simulink model "MCU_VoltLoopCal"  (R2022b)
settings: Solver=FixedStepDiscrete  StartTime=0.0  StopTime=10.0  FixedStep=0.001  RelTol=1e-3
values from neighbouring files (symbols this model uses):
  UDQ_LIMIT_ABS = 1.2    [MCU_VoltLoopCal.sldd]    (also in MCU_VoltLoopCal_objects.m = Simulink.Parameter)
  VOLTLOOP_KI = 0.1    [MCU_VoltLoopCal.sldd]    (also in MCU_VoltLoopCal_objects.m = Simulink.Parameter)
  VOLTLOOP_KP = 0.15    [MCU_VoltLoopCal.sldd]    (also in MCU_VoltLoopCal_objects.m = Simulink.Parameter)
undefined symbols (not defined in the file or in its folder): cCurrentLoopMode, cTorqueLoopMode, ParamCfg_CommandSource_u16, ParamCfg_CurrentPolarCoordinates_u16, ParamCfg_IqMax_u16, ParamCfg_MotorLsd_u16, ParamCfg_RotorFlux_u16, ParamCfg_Vc1Enable_u16, ParamCfg_VdqDest_u16, ParamCfg_WeakIdMax_u16, TESTBED
libraries: simulink x10, YS_UserDefined_Library x2
settings Model: DataDictionary=MCU_VoltLoopCal.sldd  Creator=ZYH  LastModifiedBy=ZYH
settings OptimizationCC: DefaultParameterBehavior=Inlined  EnhancedBackFolding=on  PassReuseOutputArgsAs=Individual arguments  ZeroExternalMemoryAtStartup=off  ZeroInternalMemoryAtStartup=off  OptimizeBlockOrder=speed  DifferentSizesBufferReuse=on  OptimizationCustomize=off  EfficientTunableParamExpr=on
settings DebuggingCC: ParameterTunabilityLossMsg=error
settings SFSimCC: MATLABDynamicMemAlloc=off
settings RTWCC: Description=Embedded Coder  SystemTargetFile=ert.tlc  GenCodeOnly=on  TemplateMakefile=ert_default_tmf
settings CodeAppCC: ForceParamTrailComments=on  IgnoreCustomStorageClasses=off  OperatorAnnotations=on  SimulinkDataObjDesc=on  SFDataObjDesc=on  InsertBlockDesc=on
settings ERTTargetCC: TargetLangStandard=C99 (ISO)  GenerateSampleERTMain=on  InlinedParameterPlacement=NonHierarchical  ERTCustomFileTemplate=example_file_process.tlc

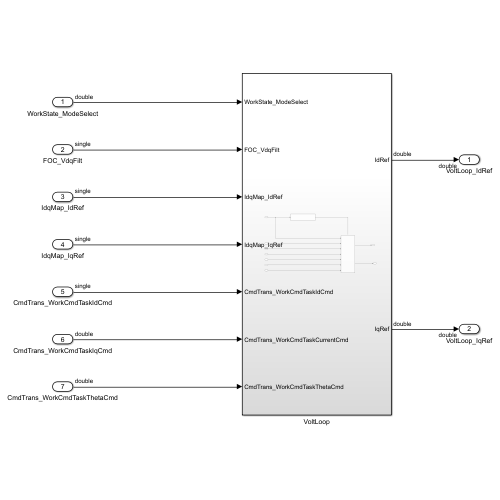
[thumbnail: Simulink's stored preview of the top-level diagram]
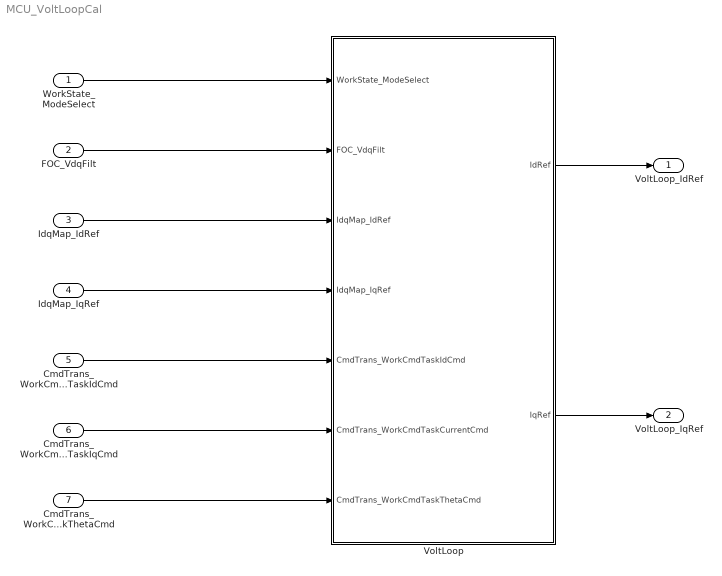
== system MCU_VoltLoopCal ==
  WorkState_ModeSelect : Inport
  FOC_VdqFilt : Inport  Port=2
  IdqMap_IdRef : Inport  Port=3
  IdqMap_IqRef : Inport  Port=4
  CmdTrans_WorkCmdTaskIdCmd : Inport  Port=5
  CmdTrans_WorkCmdTaskIqCmd : Inport  Port=6
  CmdTrans_WorkCmdTaskThetaCmd : Inport  Port=7
  VoltLoop : Subsystem
  VoltLoop_IdRef : Outport
  VoltLoop_IqRef : Outport  Port=2
  wires:
  WorkState_ModeSelect/1 -> VoltLoop/1(WorkState_ModeSelect)
  FOC_VdqFilt/1 -> VoltLoop/2(FOC_VdqFilt)
  IdqMap_IdRef/1 -> VoltLoop/3(IdqMap_IdRef)
  IdqMap_IqRef/1 -> VoltLoop/4(IdqMap_IqRef)
  CmdTrans_WorkCmdTaskIdCmd/1 -> VoltLoop/5(CmdTrans_WorkCmdTaskIdCmd)
  CmdTrans_WorkCmdTaskIqCmd/1 -> VoltLoop/6(CmdTrans_WorkCmdTaskCurrentCmd)
  CmdTrans_WorkCmdTaskThetaCmd/1 -> VoltLoop/7(CmdTrans_WorkCmdTaskThetaCmd)
  VoltLoop/1(IdRef) -> VoltLoop_IdRef/1
  VoltLoop/2(IqRef) -> VoltLoop_IqRef/1

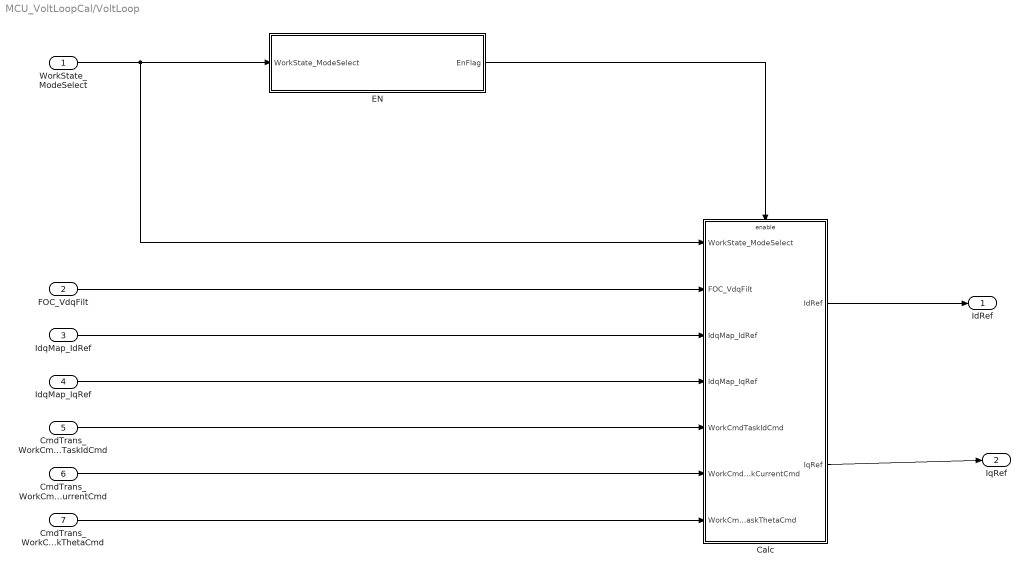
== system MCU_VoltLoopCal/VoltLoop ==
  WorkState_ModeSelect : Inport
  FOC_VdqFilt : Inport  Port=2
  IdqMap_IdRef : Inport  Port=3
  IdqMap_IqRef : Inport  Port=4
  CmdTrans_WorkCmdTaskIdCmd : Inport  Port=5
  CmdTrans_WorkCmdTaskCurrentCmd : Inport  Port=6
  CmdTrans_WorkCmdTaskThetaCmd : Inport  Port=7
  Calc : Subsystem
  EN : Subsystem
  IdRef : Outport
  IqRef : Outport  Port=2
  wires:
  WorkState_ModeSelect/1 -> Calc/1(WorkState_ModeSelect), EN/1(WorkState_ModeSelect)
  EN/1(EnFlag) -> Calc/Enable
  FOC_VdqFilt/1 -> Calc/2(FOC_VdqFilt)
  IdqMap_IdRef/1 -> Calc/3(IdqMap_IdRef)
  IdqMap_IqRef/1 -> Calc/4(IdqMap_IqRef)
  CmdTrans_WorkCmdTaskIdCmd/1 -> Calc/5(WorkCmdTaskIdCmd)
  CmdTrans_WorkCmdTaskCurrentCmd/1 -> Calc/6(WorkCmdTaskCurrentCmd)
  CmdTrans_WorkCmdTaskThetaCmd/1 -> Calc/7(WorkCmdTaskThetaCmd)
  Calc/1(IdRef) -> IdRef/1
  Calc/2(IqRef) -> IqRef/1

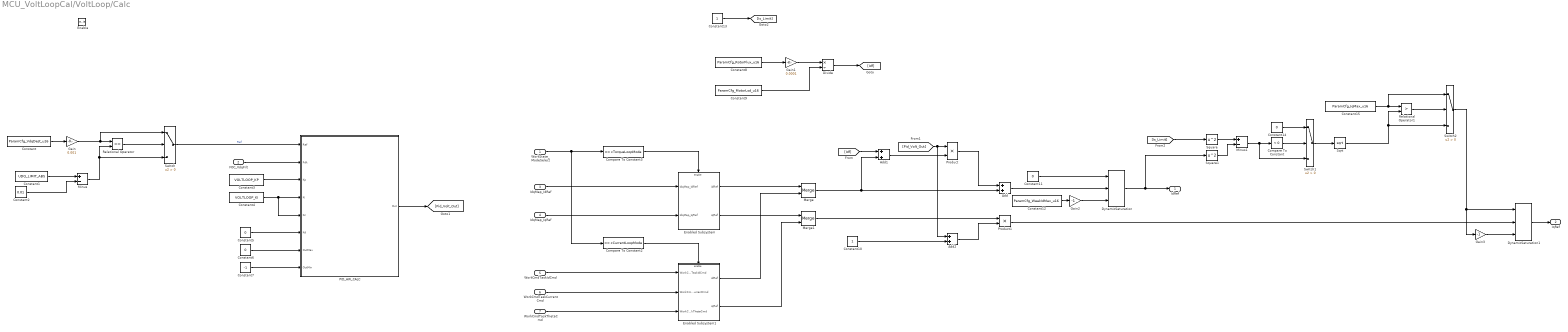
== system MCU_VoltLoopCal/VoltLoop/Calc ==
  WorkState_ModeSelect : Inport
  FOC_VdqFilt : Inport  Port=2
  IdqMap_IdRef : Inport  Port=3
  IdqMap_IqRef : Inport  Port=4
  WorkCmdTaskIdCmd : Inport  Port=5
  WorkCmdTaskCurrentCmd : Inport  Port=6
  WorkCmdTaskThetaCmd : Inport  Port=7
  Enable : EnablePort
  Add : Sum
  Add1 : Sum
  Add2 : Sum
  Compare To Constant : simulink/Logic and Bit Operations/Compare To Constant  relop=<  const=0  OutDataTypeStr=boolean
  Compare To Constant2 : simulink/Logic and Bit Operations/Compare To Constant  relop===  const=cCurrentLoopMode  OutDataTypeStr=boolean
  Compare To Constant3 : simulink/Logic and Bit Operations/Compare To Constant  relop===  const=cTorqueLoopMode  OutDataTypeStr=boolean
  Constant : Constant  Value=ParamCfg_VdqDest_u16
  Constant1 : Constant  Value=UDQ_LIMIT_ABS
  Constant10 : Constant  OutDataTypeStr=single
  Constant{5..6,11,14} (4 alike) : Constant  Value=0  OutDataTypeStr=single
  Constant12 : Constant  Value=ParamCfg_WeakIdMax_u16
  Constant13 : Constant  OutDataTypeStr=single
  Constant15 : Constant  Value=ParamCfg_IqMax_u16
  Constant2 : Constant  Value=0.01  OutDataTypeStr=single
  Constant3 : Constant  Value=VOLTLOOP_KP
  Constant4 : Constant  Value=VOLTLOOP_KI
  Constant7 : Constant  Value=-1  OutDataTypeStr=single
  Constant8 : Constant  Value=ParamCfg_RotorFlux_u16
  Constant9 : Constant  Value=ParamCfg_MotorLsd_u16
  Divide : Product  Inputs=*/
  DynamicSaturation : YS_UserDefined_Library/Saturation/DynamicSaturation
      settings: SourceProductName=YS
  DynamicSaturation1 : YS_UserDefined_Library/Saturation/DynamicSaturation
      settings: SourceProductName=YS
  Enabled Subsystem : Subsystem  TreatAsAtomicUnit=on
  Enabled Subsystem1 : Subsystem  TreatAsAtomicUnit=on
  Gain : Gain  Gain=0.001  OutDataTypeStr=single
      settings: AttributesFormatString=%<Gain>
  Gain1 : Gain  Gain=0.0001  OutDataTypeStr=single
      settings: AttributesFormatString=%<Gain>
  Gain2 : Gain  Gain=-1  ParamDataTypeStr=single  OutDataTypeStr=single
  Gain3 : Gain  Gain=-1  ParamDataTypeStr=single  OutDataTypeStr=single
  Merge : Merge
  Merge1 : Merge
  Minus : Sum  Inputs=+-
  Minus1 : Sum  Inputs=+-
  PID_AW_CALC : Subsystem
  Product : Product
  Product1 : Product
  Relational Operator : RelationalOperator  Operator=<=  OutDataTypeStr=boolean  RndMeth=Simplest  InputSameDT=off
  Relational Operator1 : RelationalOperator  Operator=>  OutDataTypeStr=boolean  RndMeth=Simplest  InputSameDT=off
  Sqrt : Sqrt
  Square : Math  Operator=square
  Square1 : Math  Operator=square
  Switch : Switch  Criteria=u2 > Threshold  SaturateOnIntegerOverflow=off  InputSameDT=off
  Switch1 : Switch  Criteria=u2 > Threshold  SaturateOnIntegerOverflow=off  InputSameDT=off
  Switch2 : Switch  Criteria=u2 > Threshold  SaturateOnIntegerOverflow=off  InputSameDT=off
  IdRef : Outport
  IqRef : Outport  Port=2
  wires:
  Constant/1 -> Gain/1
  Gain/1 -> Switch/1, Relational Operator/1
  Constant1/1 -> Minus/1
  Constant2/1 -> Minus/2
  Minus/1 -> Switch/3, Relational Operator/2
  Relational Operator/1 -> Switch/2
  Switch/1 -> PID_AW_CALC/1(Ref)  "Ref"
  FOC_VdqFilt/1 -> PID_AW_CALC/2(Fdk)
  Constant3/1 -> PID_AW_CALC/3(Kp)
  Constant4/1 -> PID_AW_CALC/5(Kc), PID_AW_CALC/4(Ki)
  Constant5/1 -> PID_AW_CALC/6(Kd)
  Constant6/1 -> PID_AW_CALC/7(OutMax)
  Constant7/1 -> PID_AW_CALC/8(OutMin)
  Compare To Constant3/1 -> Enabled Subsystem/Enable
  IdqMap_IdRef/1 -> Enabled Subsystem/1(IdqMap_IdRef)
  IdqMap_IqRef/1 -> Enabled Subsystem/2(IdqMap_IqRef)
  WorkState_ModeSelect/1 -> Compare To Constant2/1, Compare To Constant3/1
  Compare To Constant2/1 -> Enabled Subsystem1/Enable
  WorkCmdTaskIdCmd/1 -> Enabled Subsystem1/1(WorkCmdTaskIdCmd)
  WorkCmdTaskCurrentCmd/1 -> Enabled Subsystem1/2(WorkCmdTaskCurrentCmd)
  WorkCmdTaskThetaCmd/1 -> Enabled Subsystem1/3(WorkCmdTaskThetaCmd)
  Enabled Subsystem/1(idRef) -> Merge/1
  Enabled Subsystem1/1(idRef) -> Merge/2
  Enabled Subsystem/2(iqRef) -> Merge1/1
  Enabled Subsystem1/2(iqRef) -> Merge1/2
  Constant8/1 -> Gain1/1
  Gain1/1 -> Divide/1
  Constant9/1 -> Divide/2
  Divide/1 -> [Idf]
  Merge/1 -> Add1/2, Add/2
  [Idf] -> Add1/1
  PID_AW_CALC/1(Out) -> [Pid_Volt_Out]
  Add1/1 -> Product/2
  [Pid_Volt_Out] -> Add2/1, Product/1
  Product/1 -> Add/1
  Constant10/1 -> Add2/2
  Merge1/1 -> Product1/1
  Add2/1 -> Product1/2
  Add/1 -> DynamicSaturation/2
  Constant11/1 -> DynamicSaturation/1
  Constant12/1 -> Gain2/1
  Gain2/1 -> DynamicSaturation/3
  Constant13/1 -> [Is_Limit]
  [Is_Limit] -> Square/1
  Square/1 -> Minus1/1
  DynamicSaturation/1 -> IdRef/1, Square1/1
  Square1/1 -> Minus1/2
  Minus1/1 -> Switch1/3, Compare To Constant/1
  Compare To Constant/1 -> Switch1/2
  Constant14/1 -> Switch1/1
  Switch1/1 -> Sqrt/1
  Constant15/1 -> Switch2/1, Relational Operator1/1
  Sqrt/1 -> Switch2/3, Relational Operator1/2
  Relational Operator1/1 -> Switch2/2
  Product1/1 -> DynamicSaturation1/2
  Switch2/1 -> DynamicSaturation1/1, Gain3/1
  Gain3/1 -> DynamicSaturation1/3
  DynamicSaturation1/1 -> IqRef/1

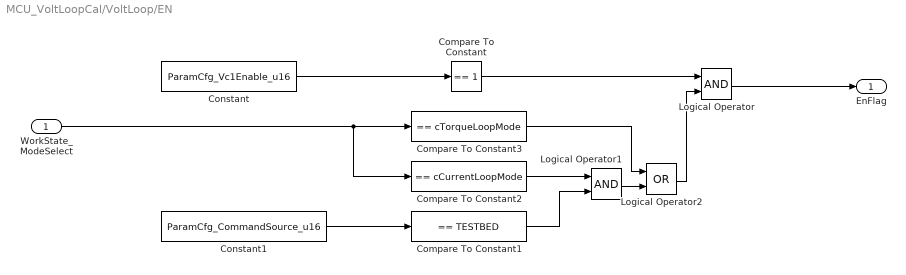
== system MCU_VoltLoopCal/VoltLoop/EN ==
  WorkState_ModeSelect : Inport
  Compare To Constant : simulink/Logic and Bit Operations/Compare To Constant  relop===  const=1  OutDataTypeStr=boolean
  Compare To Constant1 : simulink/Logic and Bit Operations/Compare To Constant  relop===  const=TESTBED  OutDataTypeStr=boolean
  Compare To Constant2 : simulink/Logic and Bit Operations/Compare To Constant  relop===  const=cCurrentLoopMode  OutDataTypeStr=boolean
  Compare To Constant3 : simulink/Logic and Bit Operations/Compare To Constant  relop===  const=cTorqueLoopMode  OutDataTypeStr=boolean
  Constant : Constant  Value=ParamCfg_Vc1Enable_u16
  Constant1 : Constant  Value=ParamCfg_CommandSource_u16
  Logical Operator : Logic  AllPortsSameDT=off  OutDataTypeStr=boolean
  Logical Operator1 : Logic  AllPortsSameDT=off  OutDataTypeStr=boolean
  Logical Operator2 : Logic  Operator=OR  AllPortsSameDT=off  OutDataTypeStr=boolean
  EnFlag : Outport
  wires:
  Compare To Constant/1 -> Logical Operator/1
  Logical Operator2/1 -> Logical Operator/2
  Compare To Constant3/1 -> Logical Operator2/1
  WorkState_ModeSelect/1 -> Compare To Constant2/1, Compare To Constant3/1
  Compare To Constant1/1 -> Logical Operator1/2
  Constant/1 -> Compare To Constant/1
  Constant1/1 -> Compare To Constant1/1
  Logical Operator1/1 -> Logical Operator2/2
  Compare To Constant2/1 -> Logical Operator1/1
  Logical Operator/1 -> EnFlag/1

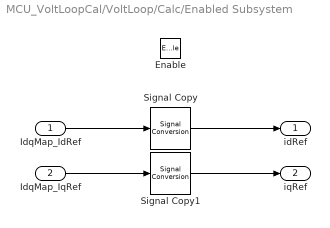
== system MCU_VoltLoopCal/VoltLoop/Calc/Enabled Subsystem ==
  IdqMap_IdRef : Inport
  IdqMap_IqRef : Inport  Port=2
  Enable : EnablePort
  Signal Copy : SignalConversion  OverrideOpt=off
  Signal Copy1 : SignalConversion  OverrideOpt=off
  idRef : Outport
  iqRef : Outport  Port=2
  wires:
  IdqMap_IdRef/1 -> Signal Copy/1
  IdqMap_IqRef/1 -> Signal Copy1/1
  Signal Copy/1 -> idRef/1
  Signal Copy1/1 -> iqRef/1

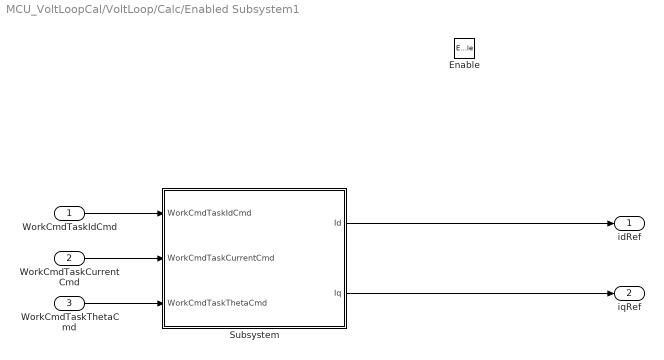
== system MCU_VoltLoopCal/VoltLoop/Calc/Enabled Subsystem1 ==
  WorkCmdTaskIdCmd : Inport
  WorkCmdTaskCurrentCmd : Inport  Port=2
  WorkCmdTaskThetaCmd : Inport  Port=3
  Enable : EnablePort
  Subsystem : Subsystem
  idRef : Outport
  iqRef : Outport  Port=2
  wires:
  WorkCmdTaskIdCmd/1 -> Subsystem/1(WorkCmdTaskIdCmd)
  WorkCmdTaskCurrentCmd/1 -> Subsystem/2(WorkCmdTaskCurrentCmd)
  WorkCmdTaskThetaCmd/1 -> Subsystem/3(WorkCmdTaskThetaCmd)
  Subsystem/1(Id) -> idRef/1
  Subsystem/2(Iq) -> iqRef/1

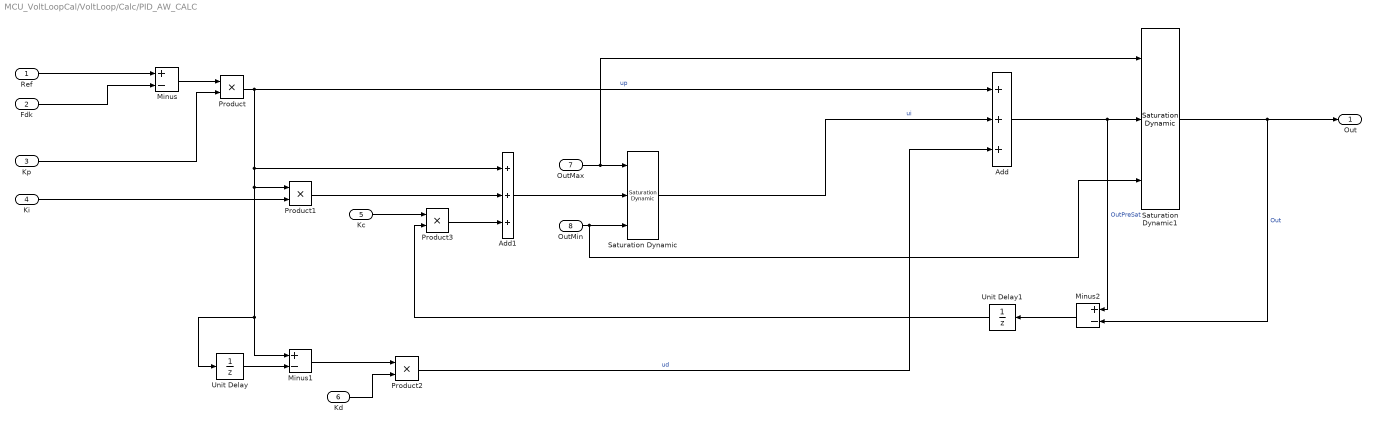
== system MCU_VoltLoopCal/VoltLoop/Calc/PID_AW_CALC ==
  Ref : Inport
  Fdk : Inport  Port=2
  Kp : Inport  Port=3
  Ki : Inport  Port=4
  Kc : Inport  Port=5
  Kd : Inport  Port=6
  OutMax : Inport  Port=7
  OutMin : Inport  Port=8
  Add : Sum  Inputs=+++
  Add1 : Sum  Inputs=+++
  Minus : Sum  Inputs=+-
  Minus1 : Sum  Inputs=+-
  Minus2 : Sum  Inputs=+-
  Product{,1..3} (4 alike) : Product
  Saturation Dynamic : simulink/Discontinuities/Saturation Dynamic  OutMin=[]  OutMax=[]  OutDataTypeStr=Inherit: Same as second input  OutDataType=fixdt(1, 16)  OutScaling=2^-10  DoSatur=off
  Saturation Dynamic1 : simulink/Discontinuities/Saturation Dynamic  OutMin=[]  OutMax=[]  OutDataTypeStr=Inherit: Same as second input  OutDataType=fixdt(1, 16)  OutScaling=2^-10  DoSatur=off
  Unit Delay : UnitDelay  SampleTime=-1  HasFrameUpgradeWarning=on
  Unit Delay1 : UnitDelay  SampleTime=-1  HasFrameUpgradeWarning=on
  Out : Outport
  wires:
  Ref/1 -> Minus/1
  Fdk/1 -> Minus/2
  Minus/1 -> Product/1
  Kp/1 -> Product/2
  Product/1 -> Add1/1, Unit Delay/1, Minus1/1, Product1/1, Add/1  "up"
  Ki/1 -> Product1/2
  Add/1 -> Minus2/1, Saturation Dynamic1/2  "OutPreSat"
  Product1/1 -> Add1/2
  OutMax/1 -> Saturation Dynamic1/1, Saturation Dynamic/1
  Add1/1 -> Saturation Dynamic/2
  OutMin/1 -> Saturation Dynamic1/3, Saturation Dynamic/3
  Saturation Dynamic/1 -> Add/2  "ui"
  Minus1/1 -> Product2/1
  Kd/1 -> Product2/2
  Product2/1 -> Add/3  "ud"
  Saturation Dynamic1/1 -> Minus2/2, Out/1  "Out"
  Unit Delay/1 -> Minus1/2
  Minus2/1 -> Unit Delay1/1
  Product3/1 -> Add1/3
  Kc/1 -> Product3/1
  Unit Delay1/1 -> Product3/2

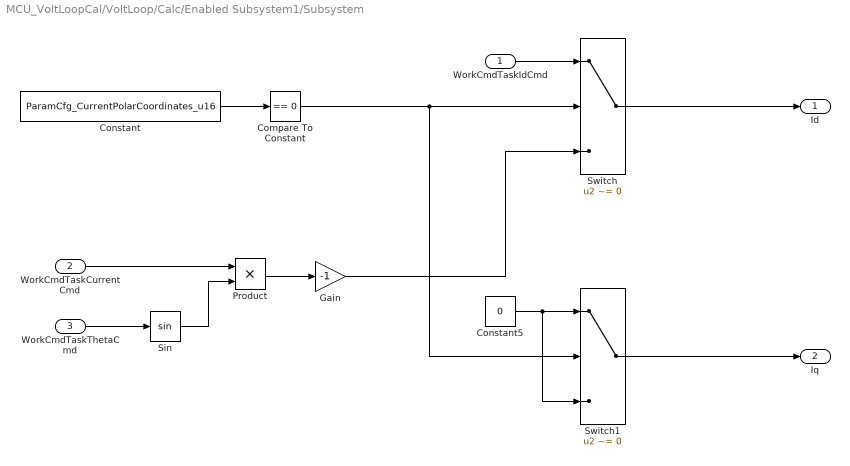
== system MCU_VoltLoopCal/VoltLoop/Calc/Enabled Subsystem1/Subsystem ==
  WorkCmdTaskIdCmd : Inport
  WorkCmdTaskCurrentCmd : Inport  Port=2
  WorkCmdTaskThetaCmd : Inport  Port=3
  Compare To Constant : simulink/Logic and Bit Operations/Compare To Constant  relop===  const=0  OutDataTypeStr=boolean
  Constant : Constant  Value=ParamCfg_CurrentPolarCoordinates_u16
  Constant5 : Constant  Value=0  OutDataTypeStr=single
  Gain : Gain  Gain=-1  OutDataTypeStr=single
  Product : Product
  Sin : Trigonometry
  Switch : Switch  Criteria=u2 ~= 0  SaturateOnIntegerOverflow=off  InputSameDT=off
  Switch1 : Switch  Criteria=u2 ~= 0  SaturateOnIntegerOverflow=off  InputSameDT=off
  Id : Outport
  Iq : Outport  Port=2
  wires:
  Constant/1 -> Compare To Constant/1
  Compare To Constant/1 -> Switch1/2, Switch/2
  Switch1/1 -> Iq/1
  Switch/1 -> Id/1
  WorkCmdTaskIdCmd/1 -> Switch/1
  Constant5/1 -> Switch1/3, Switch1/1
  WorkCmdTaskThetaCmd/1 -> Sin/1
  WorkCmdTaskCurrentCmd/1 -> Product/1
  Sin/1 -> Product/2
  Product/1 -> Gain/1
  Gain/1 -> Switch/3
